simulink model "three_phase_Gen_SpeedControl_2023A"  (R2023a)
settings: Solver=VariableStepAuto  StartTime=0.0  StopTime=10.0  RelTol=1e-3
values from neighbouring files (symbols this model uses):
  Ts = T_pwm    (= 5e-05)    [FOC_Param.m]    (also in FOC_simulationParameters.m; mcb_pmsm_fwc_qep_f28379d_data.m; open_loop_control_script.m = T_pwm)
undefined symbols (not defined in the file or in its folder): rated
libraries: mcbcontrolslib x2
settings Model: Creator=ela19kfs  LastModifiedBy=ela19kfs

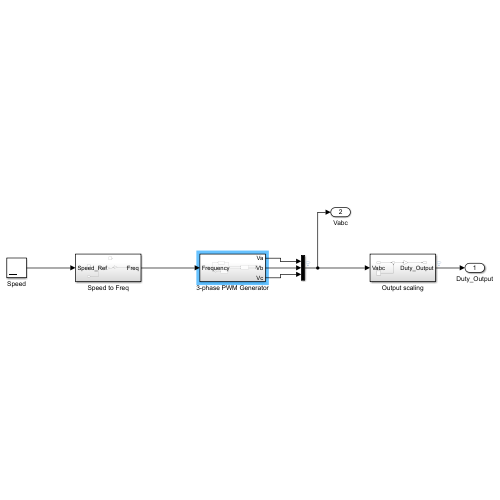
[thumbnail: Simulink's stored preview of the top-level diagram]
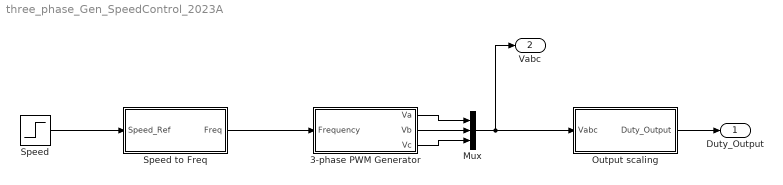
== system three_phase_Gen_SpeedControl_2023A ==
  3-phase PWM Generator : Subsystem
  Mux : Mux  Inputs=3
  Output scaling : Subsystem
  Speed : Step  SampleTime=0
  Speed to Freq : Subsystem
  Duty_Output : Outport
  Vabc : Outport  Port=2
  wires:
  Speed/1 -> Speed to Freq/1(Speed_Ref)
  Speed to Freq/1(Freq) -> 3-phase PWM Generator/1(Frequency)
  3-phase PWM Generator/1(Va) -> Mux/1
  3-phase PWM Generator/2(Vb) -> Mux/2
  3-phase PWM Generator/3(Vc) -> Mux/3
  Mux/1 -> Output scaling/1(Vabc), Vabc/1
  Output scaling/1(Duty_Output) -> Duty_Output/1

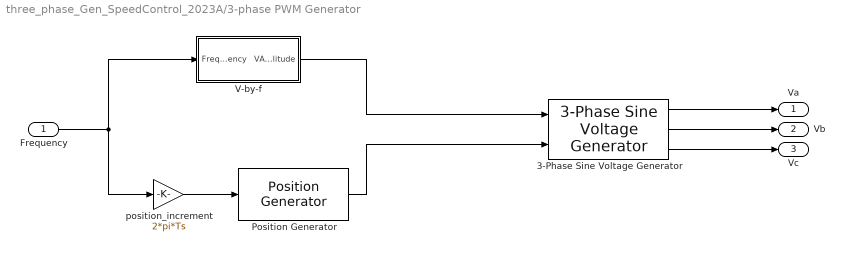
== system three_phase_Gen_SpeedControl_2023A/3-phase PWM Generator ==
  Frequency : Inport
  3-Phase Sine Voltage Generator : mcbcontrolslib/3-Phase Sine Voltage Generator  AngleInput=Radians  N_points=1024
  Position Generator : mcbcontrolslib/Position Generator  AngleOutput=Radians  ExternalReset=none  Offset=0
  V-by-f : Subsystem
  position_increment : Gain  Gain=2*pi*Ts  RndMeth=Simplest  OutDataTypeStr=Inherit: Same as input
  Va : Outport
  Vb : Outport  Port=2
  Vc : Outport  Port=3
  wires:
  V-by-f/1(VAmplitude) -> 3-Phase Sine Voltage Generator/1
  3-Phase Sine Voltage Generator/3 -> Vc/1
  position_increment/1 -> Position Generator/1
  3-Phase Sine Voltage Generator/1 -> Va/1
  3-Phase Sine Voltage Generator/2 -> Vb/1
  Frequency/1 -> V-by-f/1(Frequency), position_increment/1
  Position Generator/1 -> 3-Phase Sine Voltage Generator/2

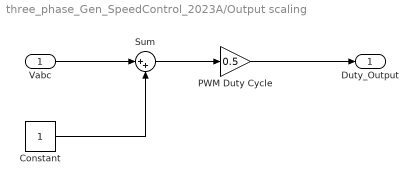
== system three_phase_Gen_SpeedControl_2023A/Output scaling ==
  Vabc : Inport
  Constant : Constant
  PWM Duty Cycle : Gain  Gain=0.5
  Sum : Sum  Inputs=|++
  Duty_Output : Outport
  wires:
  Vabc/1 -> Sum/1
  Constant/1 -> Sum/2
  Sum/1 -> PWM Duty Cycle/1
  PWM Duty Cycle/1 -> Duty_Output/1

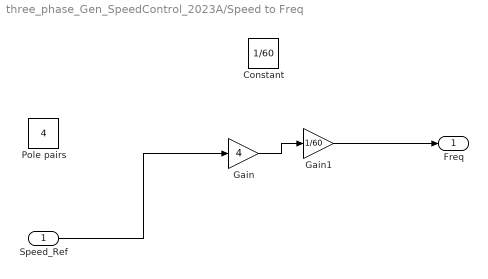
== system three_phase_Gen_SpeedControl_2023A/Speed to Freq ==
  Speed_Ref : Inport
  Constant : Constant  Value=1/60
  Gain : Gain  Gain=4
  Gain1 : Gain  Gain=1/60
  Pole pairs : Constant  Value=4
  Freq : Outport
  wires:
  Speed_Ref/1 -> Gain/1
  Gain1/1 -> Freq/1
  Gain/1 -> Gain1/1

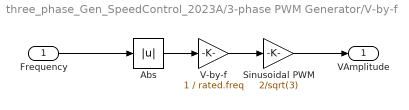
== system three_phase_Gen_SpeedControl_2023A/3-phase PWM Generator/V-by-f ==
  Frequency : Inport
  Abs : Abs  RndMeth=Simplest  SaturateOnIntegerOverflow=off
  Sinusoidal PWM : Gain  Gain=2/sqrt(3)  RndMeth=Simplest  OutDataTypeStr=Inherit: Same as input
  V-by-f : Gain  Gain=1 / rated.freq  RndMeth=Simplest  OutDataTypeStr=Inherit: Same as input
  VAmplitude : Outport
  wires:
  Abs/1 -> V-by-f/1
  V-by-f/1 -> Sinusoidal PWM/1
  Frequency/1 -> Abs/1
  Sinusoidal PWM/1 -> VAmplitude/1
